simulink model "Meshsin"  (Simulink 3.00)
settings: Solver=ode45  StartTime=0.0  StopTime=5  RelTol=1e-3
values from neighbouring files (symbols this model uses):
  x10 = 0    [v515.m]    (also in v516.m; v517.m)
  x20 = 0    [v515.m]    (also in v516.m; v517.m)

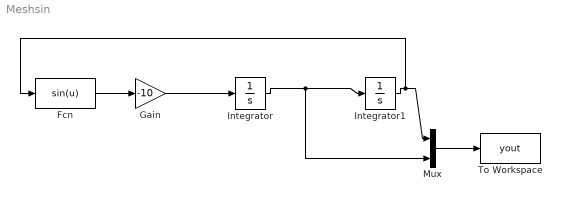
== system Meshsin ==
  Fcn : Fcn  Expr=sin(u)
  Gain : Gain  Gain=-10  SaturateOnIntegerOverflow=on
  Integrator : Integrator  ExternalReset=none  InitialConditionSource=internal  InitialCondition=x20  LimitOutput=off  UpperSaturationLimit=inf  LowerSaturationLimit=-inf  ShowSaturationPort=off  ShowStatePort=off  AbsoluteTolerance=auto
  Integrator1 : Integrator  ExternalReset=none  InitialConditionSource=internal  InitialCondition=x10  LimitOutput=off  UpperSaturationLimit=inf  LowerSaturationLimit=-inf  ShowSaturationPort=off  ShowStatePort=off  AbsoluteTolerance=auto
  Mux : Mux  Inputs=2
  To Workspace : ToWorkspace  VariableName=yout  SampleTime=-1  SaveFormat=Matrix
  wires:
  Integrator/1 -> Integrator1/1, Mux/2
  Mux/1 -> To Workspace/1
  Integrator1/1 -> Mux/1, Fcn/1
  Fcn/1 -> Gain/1
  Gain/1 -> Integrator/1
